simulink model "integrator_MRFT_control_SOIPTD"  (R2019b)
settings: Solver=ode2  StartTime=0.0  StopTime=10.0  FixedStep=0.001  RelTol=1e-3
undefined symbols (not defined in the file or in its folder): h_ref, K, Ki, T1, T2, tau, v_ref
libraries: simulink x3
settings Model: Creator=Ayyad  LastModifiedBy=aaa_b
settings DataIOCC: ReturnWorkspaceOutputs=off
settings DebuggingCC: ArithmeticOperatorsInVariantConditions=warning
settings SFSimCC: SimUseLocalCustomCode=off  CustomCodeUndefinedFunction=UseInterfaceOnly
settings RTWCC: RTWUseLocalCustomCode=off

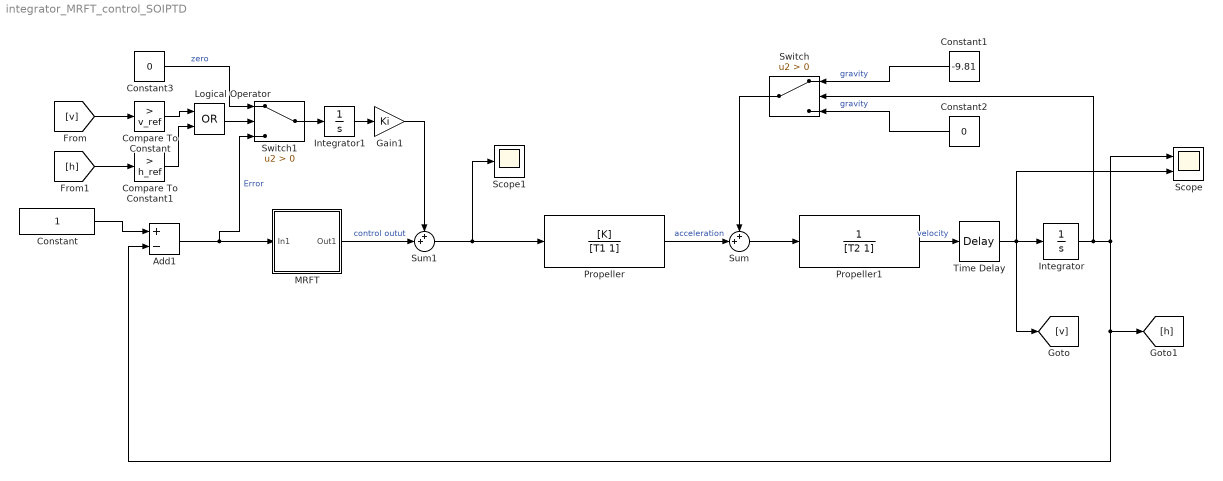
== system integrator_MRFT_control_SOIPTD ==
  Add1 : Sum  Inputs=+-
  Compare To Constant : simulink/Logic and Bit Operations/Compare To Constant  relop=>  const=v_ref  OutDataTypeStr=boolean
  Compare To Constant1 : simulink/Logic and Bit Operations/Compare To Constant  relop=>  const=h_ref  OutDataTypeStr=boolean
  Constant : Constant
  Constant1 : Constant  Value=-9.81
  Constant2 : Constant  Value=0
  Constant3 : Constant  Value=0
  Gain1 : Gain  Gain=Ki
  Integrator : Integrator  LimitOutput=on  LowerSaturationLimit=0
  Integrator1 : Integrator
  Logical Operator : Logic  Operator=OR  AllPortsSameDT=off  OutDataTypeStr=boolean
  MRFT : Subsystem
  Propeller : TransferFcn  Numerator=[K]  Denominator=[T1 1]
  Propeller1 : TransferFcn  Denominator=[T2 1]
  Scope : Scope  NumInputPorts=2
  Scope1 : Scope
  Sum : Sum  Inputs=++|
  Sum1 : Sum  Inputs=++|
  Switch : Switch  Criteria=u2 > Threshold
  Switch1 : Switch  Criteria=u2 > Threshold
  Time Delay : TransportDelay  DelayTime=tau
  wires:
  Propeller/1 -> Sum/2  "acceleration"
  Sum1/1 -> Propeller/1, Scope1/1
  Integrator/1 -> Switch/2, [h], Add1/2, Scope/1
  MRFT/1(Out1) -> Sum1/2  "control outut"
  Add1/1 -> Switch1/3, MRFT/1(In1)  "Error"
  Constant/1 -> Add1/1
  Sum/1 -> Propeller1/1
  Switch/1 -> Sum/1
  Constant1/1 -> Switch/1  "gravity"
  Constant2/1 -> Switch/3  "gravity"
  Switch1/1 -> Integrator1/1
  Constant3/1 -> Switch1/1  "zero"
  [v] -> Compare To Constant/1
  Integrator1/1 -> Gain1/1
  Gain1/1 -> Sum1/1
  [h] -> Compare To Constant1/1
  Compare To Constant1/1 -> Logical Operator/2
  Compare To Constant/1 -> Logical Operator/1
  Logical Operator/1 -> Switch1/2
  Propeller1/1 -> Time Delay/1  "velocity"
  Time Delay/1 -> Scope/2, [v], Integrator/1

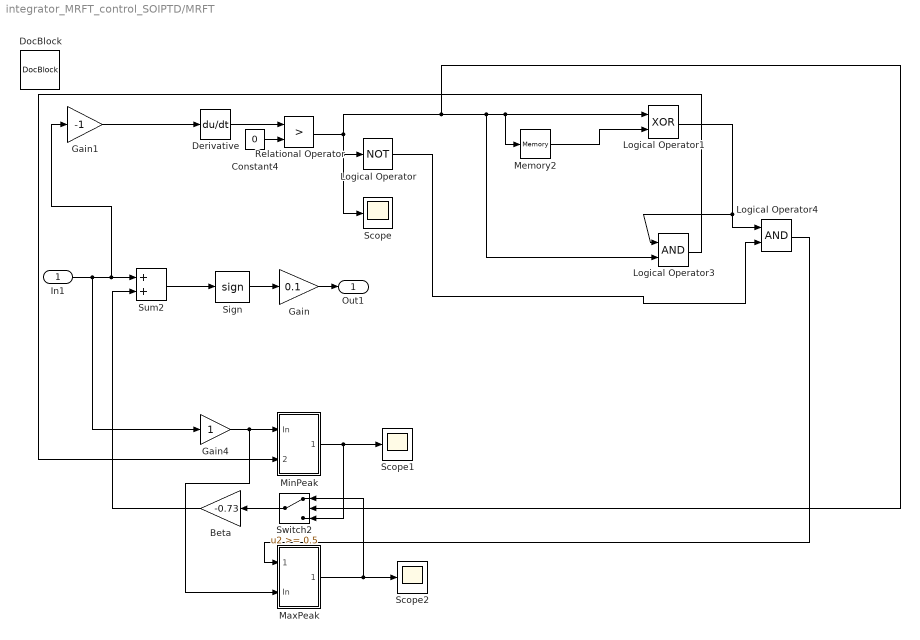
== system integrator_MRFT_control_SOIPTD/MRFT ==
  In1 : Inport
  Beta : Gain  Gain=-0.73  SaturateOnIntegerOverflow=on  OutDataTypeStr=Inherit: Same as input  ParamDataTypeStr=Inherit: Same as input
  Constant4 : Constant  Value=0
  Derivative : Derivative  CoefficientInTFapproximation=0
  DocBlock : simulink/Model-Wide Utilities/DocBlock  DocumentType=Text
      content=|
      | UserData_79
  Gain : Gain  Gain=0.1  SaturateOnIntegerOverflow=on  OutDataTypeStr=Inherit: Same as input  ParamDataTypeStr=Inherit: Same as input
  Gain1 : Gain  Gain=-1  SaturateOnIntegerOverflow=on  OutDataTypeStr=Inherit: Same as input  ParamDataTypeStr=Inherit: Same as input
  Gain4 : Gain  SaturateOnIntegerOverflow=on  OutDataTypeStr=Inherit: Same as input  ParamDataTypeStr=Inherit: Same as input
  Logical Operator : Logic  Operator=NOT  Inputs=1
  Logical Operator1 : Logic  Operator=XOR
  Logical Operator3 : Logic
  Logical Operator4 : Logic
  MaxPeak : Subsystem
  Memory2 : Memory
  MinPeak : Subsystem
  Relational Operator : RelationalOperator  Operator=>  RndMeth=Nearest  InputSameDT=on
  Scope : Scope
  Scope1 : Scope
  Scope2 : Scope
  Sign : Signum
  Sum2 : Sum  SaturateOnIntegerOverflow=on  InputSameDT=on  OutDataTypeStr=Inherit: Same as first input
  Switch2 : Switch  Threshold=0.5  SaturateOnIntegerOverflow=on  InputSameDT=on
  Out1 : Outport  VectorParamsAs1DForOutWhenUnconnected=off
  wires:
  Gain1/1 -> Derivative/1
  Memory2/1 -> Logical Operator1/2
  In1/1 -> Sum2/1, Gain1/1, Gain4/1
  Gain/1 -> Out1/1
  Derivative/1 -> Relational Operator/1
  MinPeak/1(Out) -> Switch2/3, Scope1/1
  MaxPeak/1(Out) -> Switch2/1, Scope2/1
  Beta/1 -> Sum2/2
  Sum2/1 -> Sign/1
  Gain4/1 -> MaxPeak/2(In), MinPeak/1(In)
  Sign/1 -> Gain/1
  Logical Operator/1 -> Logical Operator4/2
  Logical Operator3/1 -> MinPeak/2(Cntrl)
  Relational Operator/1 -> Switch2/2, Logical Operator3/2, Memory2/1, Logical Operator1/1, Logical Operator/1, Scope/1
  Constant4/1 -> Relational Operator/2
  Logical Operator4/1 -> MaxPeak/1(Cntrl)
  Logical Operator1/1 -> Logical Operator3/1, Logical Operator4/1
  Switch2/1 -> Beta/1

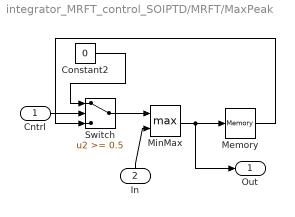
== system integrator_MRFT_control_SOIPTD/MRFT/MaxPeak ==
  Cntrl : Inport
  In : Inport  Port=2
  Constant2 : Constant  Value=0
  Memory : Memory
  MinMax : MinMax  Function=max  Inputs=2  SaturateOnIntegerOverflow=on  InputSameDT=on
  Switch : Switch  Threshold=0.5  SaturateOnIntegerOverflow=on  InputSameDT=on
  Out : Outport  VectorParamsAs1DForOutWhenUnconnected=off
  wires:
  Cntrl/1 -> Switch/2
  In/1 -> MinMax/2
  Memory/1 -> Switch/3
  Constant2/1 -> Switch/1
  Switch/1 -> MinMax/1
  MinMax/1 -> Out/1, Memory/1

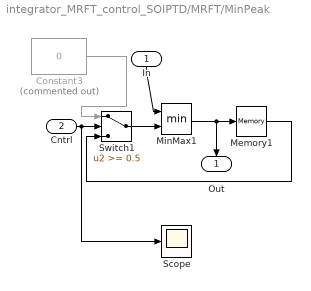
== system integrator_MRFT_control_SOIPTD/MRFT/MinPeak ==
  In : Inport
  Cntrl : Inport  Port=2
  Constant3 : Constant  Commented=on  Value=0
  Memory1 : Memory
  MinMax1 : MinMax  Inputs=2  SaturateOnIntegerOverflow=on  InputSameDT=on
  Scope : Scope
  Switch1 : Switch  Threshold=0.5  SaturateOnIntegerOverflow=on  InputSameDT=on
  Out : Outport  VectorParamsAs1DForOutWhenUnconnected=off
  wires:
  Cntrl/1 -> Scope/1, Switch1/2
  In/1 -> MinMax1/1
  Constant3/1 -> Switch1/1
  Memory1/1 -> Switch1/3
  Switch1/1 -> MinMax1/2
  MinMax1/1 -> Out/1, Memory1/1
